simulink model "mdaqdemo_vs"  (R2013a)
settings: Solver=FixedStepDiscrete  StartTime=0.0  StopTime=inf  RelTol=1e-3
PreLoadFcn:
  | template_orig = fliplr([109 100]);
  | template_size = fliplr([18 22]);
  | search_border = fliplr([10 15]);
  | pos.template_orig = fliplr(template_orig);
  | pos.template_size = template_size;
  | pos.search_border = search_border;
  | pos.template_center = floor((template_size-1)/2);
  | pos.template_center_pos = pos.template_orig + ...
  |     pos.template_center - 1;
undefined symbols (not defined in the file or in its folder): gray
libraries: visiontextngfix x3, visionsinks x2, visiongeotforms x1, dspvision x1
Description:
  | Image stabilization demo.
settings Model: Tag="0  0  0  0  0  1"  FPTRunName=Active  ExtModeAutoUpdateStatusClock=off  Creator=The MathWorks Inc.  LastModifiedBy=witczenko
settings DataIOCC: SignalLoggingSaveFormat=ModelDataLogs  SaveOutput=off  SaveTime=off  SignalLoggingName=logsOut
settings OptimizationCC: InlineParams=on  ExpressionDepthLimit=2147483647  InitFltsAndDblsToZero=on  OptimizeModelRefInitCode=on  LifeSpan=Inf  BufferReusableBoundary=off
settings DebuggingCC: CheckExecutionContextPreStartOutputMsg=on  CheckExecutionContextRuntimeOutputMsg=on  SolverPrmCheckMsg=none  InheritedTsInSrcMsg=none  MultiTaskDSMMsg=warning  SigSpecEnsureSampleTimeMsg=none  ParameterPrecisionLossMsg=none  UnderSpecifiedDataTypeMsg=error  FcnCallInpInsideContextMsg=EnableAllAsWarning  FrameProcessingCompatibilityMsg=error  BusObjectLabelMismatch=none
settings HardwareCC: ProdBitPerLong=40  ProdLargestAtomicInteger=Integer  ProdIntDivRoundTo=Zero  ProdEndianess=LittleEndian  ProdHWDeviceType=Texas Instruments->C6000  TargetBitPerPointer=64  TargetLongLongMode=on  TargetIntDivRoundTo=Zero  TargetEndianess=LittleEndian  TargetWordSize=64  TargetHWDeviceType=MATLAB Host  ProdEqTarget=off
settings ModelReferenceCC: UpdateModelReferenceTargets=IfOutOfDate
settings RTWCC: SystemTargetFile=microdaq.tlc  TemplateMakefile=microdaq.tmf  PostCodeGenCommand=microdaq_postcodegen(buildInfo)  Description=MicroDAQ Real-Time Measurement System
settings CodeAppCC: IgnoreCustomStorageClasses=off
settings STFCustomTargetCC: CodeReplacementLibrary=C89/C90 (ANSI)  CombineOutputUpdateFcns=on  ERTCustomFileBanners=on  SupportContinuousTime=off  SupportNonInlinedSFcns=off  MATLABClassNameForMDSCustomization=Simulink.SoftwareTarget.ERTCustomization  SystemTargetFile=microdaq.tlc
settings ERTTargetCC: CodeReplacementLibrary=C89/C90 (ANSI)  GenerateSampleERTMain=off  ParMdlRefBuildCompliant=off  CompOptLevelCompliant=off  ConcurrentExecutionCompliant=off  ERTFirstTimeCompliant=off  ModelStepFunctionPrototypeControlCompliant=off  CPPClassGenCompliant=off  ERTCustomFileTemplate=microdaq_main.tlc

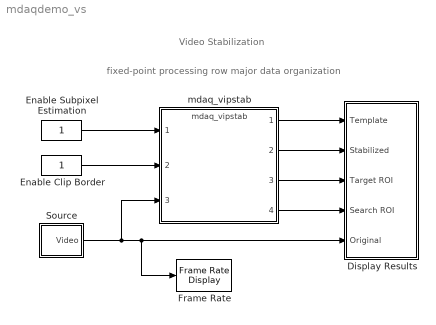
== system mdaqdemo_vs ==
  note: Video Stabilization
  note: fixed-point processing
      | row major data organization
  Display Results : Subsystem
  Enable Clip Border : Constant  VectorParams1D=off  OutDataTypeStr=boolean  SampleTime=-1
  Enable Subpixel Estimation : Constant  VectorParams1D=off  OutDataTypeStr=boolean  SampleTime=-1
  Frame Rate : visionsinks/Frame Rate Display  UpdateRate=10
  Source : Subsystem
  mdaq_vipstab : ModelReference  ModelNameDialog=mdaq_vipstab  SimulationMode=Processor-in-the-loop (PIL)  ModelReferenceVersion=1.1886
  wires:
  Source/1(Video) -> mdaq_vipstab/3, Frame Rate/1, Display Results/5(Original)
  mdaq_vipstab/1 -> Display Results/1(Template)
  mdaq_vipstab/2 -> Display Results/2(Stabilized)
  Enable Subpixel Estimation/1 -> mdaq_vipstab/1
  Enable Clip Border/1 -> mdaq_vipstab/2
  mdaq_vipstab/3 -> Display Results/3(Target ROI)
  mdaq_vipstab/4 -> Display Results/4(Search ROI)

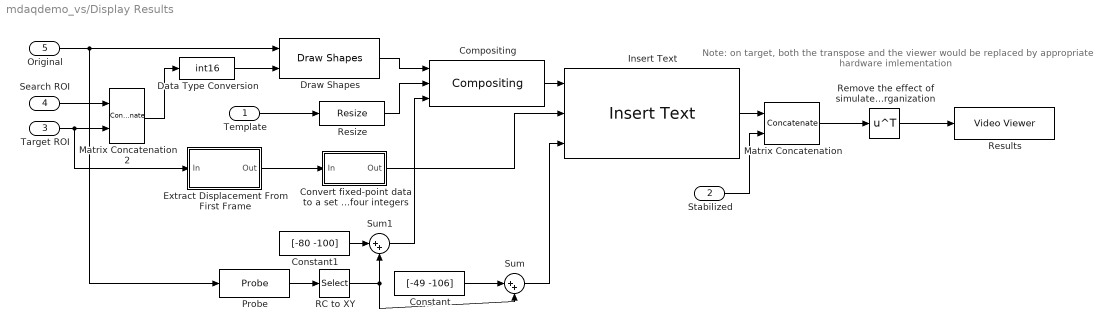
== system mdaqdemo_vs/Display Results ==
  note: Note: on target, both the transpose and the viewer
      | would be replaced by appropriate hardware imlementation
  Template : Inport
  Stabilized : Inport  Port=2
  Target ROI : Inport  Port=3
  Search ROI : Inport  Port=4
  Original : Inport  Port=5
  Compositing : visiontextngfix/Compositing  operation=Binary mask  bFacSrc=Specify via dialog  mFacSrc=Specify via dialog  bFactor=1  mFactor=1  source=Input port  coordinates=[160 220]  prodOutputMode=Binary point scaling  prodOutputWordLength=32  prodOutputFracLength=10  roundingMode=Floor  overflowMode=off
  Constant : Constant  Value=[-49 -106]  OutDataTypeStr=int16
  Constant1 : Constant  Value=[-80 -100]  OutDataTypeStr=int16
  Convert fixed-point data to a set of four integers : Subsystem
  Data Type Conversion : DataTypeConversion  OutDataTypeStr=int16
  Draw Shapes : visiontextngfix/Draw Shapes  shape=Rectangles  fill=off  fillClrSource=Specify via dialog  display=White  intensity=200  color=[200 255 100]  opacity=0.6  viewport=Entire image  antialiasing=off  inType=Intensity  imagePorts=One multidimensional signal  prodOutputMode=Binary point scaling  prodOutputWordLength=32  prodOutputFracLength=14  memoryMode=Specify word length  memoryWordLength=16  memoryFracLength=15  roundingMode=Floor  overflowMode=off
  Extract Displacement From First Frame : Subsystem
  Insert Text : visiontextngfix/Insert Text  inputType=Obsolete  theText='(%+03d.%02d,%+03d.%02d)'  fontFace=LucidaTypewriterRegular  dummyVar1=0  blockFontSize=14  antiAliased=on  getTextLocFrom=Input port  textLoc=[214 191]  getTextColorFrom=Specify via dialog  textColor=255  getTextIntensityFrom=Specify via dialog  textIntensity=255  getTextOpacityFrom=Specify via dialog  textOpacity=1.0  dummyVar2=0  dummyVar3=0  dummyVar4=0  imagePorts=One multidimensional signal  isInputTransposed=on
  Matrix Concatenation : Concatenate  Mode=Multidimensional array
  Matrix Concatenation2 : Concatenate  Mode=Multidimensional array
  Probe : Probe  ProbeWidth=off  ProbeSampleTime=off  ProbeComplexSignal=off  ProbeSignalDimensions=on  ProbeDimensionsDataType=int16
  RC to XY : Selector  IndexOptions=Index vector (dialog)  Indices=[2 1]  OutputSizes=1
  Remove the effect of simulated row major data organization : Math  Operator=transpose  SaturateOnIntegerOverflow=on
  Resize : visiongeotforms/Resize  specify=Output size as a percentage of input size  rfactor=300  outCols=25  outRows=25  outRowsCols=[25 35]  interp_method=Nearest neighbor  antialias=off  useROI=off  roiFlag=off  prodOutputMode=Binary point scaling  prodOutputWordLength=32  prodOutputFracLength=10  roundingMode=Nearest  overflowMode=on
  Results : visionsinks/Video Viewer  inputType=Obsolete7b  imagePorts=One multidimensional signal  useColorMap=off  colormapValue=gray(256)  specRange=off  minInputVal=0  maxInputVal=255  FigPos=[97 364 640 263]  AxisZoom=on  trueSizedOnce=on  OpenAtMdlStart=on  DefaultConfigurationName=vipscopes.VideoViewerScopeCfg
  Sum : Sum  Inputs=|++
  Sum1 : Sum  Inputs=|++
  wires:
  Remove the effect of simulated row major data organization/1 -> Results/1
  RC to XY/1 -> Sum/2, Sum1/2
  Constant/1 -> Sum/1
  Sum/1 -> Insert Text/3
  Probe/1 -> RC to XY/1
  Sum1/1 -> Compositing/3
  Constant1/1 -> Sum1/1
  Template/1 -> Resize/1
  Compositing/1 -> Insert Text/1
  Insert Text/1 -> Matrix Concatenation/1
  Resize/1 -> Compositing/2
  Stabilized/1 -> Matrix Concatenation/2
  Draw Shapes/1 -> Compositing/1
  Matrix Concatenation/1 -> Remove the effect of simulated row major data organization/1
  Convert fixed-point data to a set of four integers/1(Out) -> Insert Text/2
  Matrix Concatenation2/1 -> Data Type Conversion/1
  Original/1 -> Probe/1, Draw Shapes/1
  Extract Displacement From First Frame/1(Out) -> Convert fixed-point data to a set of four integers/1(In)
  Search ROI/1 -> Matrix Concatenation2/1
  Target ROI/1 -> Matrix Concatenation2/2, Extract Displacement From First Frame/1(In)
  Data Type Conversion/1 -> Draw Shapes/2

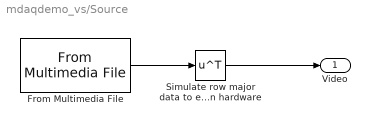
== system mdaqdemo_vs/Source ==
  From Multimedia File : dspvision/From Multimedia File  inputFilename=shaky_car.avi  loop=on  numPlays=inf  outputStreams=Video and audio  videoDataType=uint8  audioDataType=int16  inheritSampleTime=on  userDefinedSampleTime=1/30  noAudioOutput=off  isIntensityVideo=off  fourcc=Intensity  colorVideoFormat=Separate color signals  outputEOF=off  dataOrg=Column-major  audioFrameSize=1024  computeAudioFrameSize=off  outSamplingMode=Frame based
  Simulate row major data to ease implementation on hardware : Math  Operator=transpose  SaturateOnIntegerOverflow=on
  Video : Outport
  wires:
  Simulate row major data to ease implementation on hardware/1 -> Video/1
  From Multimedia File/1 -> Simulate row major data to ease implementation on hardware/1

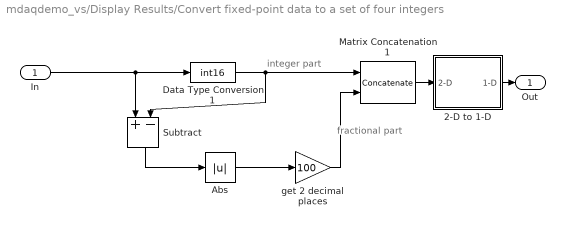
== system mdaqdemo_vs/Display Results/Convert fixed-point data to a set of four integers ==
  note: integer part
  note: fractional
      | part
  In : Inport
  2-D to 1-D : Subsystem
  Abs : Abs
  Data Type Conversion1 : DataTypeConversion  OutDataTypeStr=int16  RndMeth=Zero
  Matrix Concatenation1 : Concatenate  Mode=Multidimensional array
  Subtract : Sum  Inputs=+-  OutDataTypeStr=Inherit: Same as first input
  get 2 decimal places : Gain  Gain=100  OutDataTypeStr=fixdt(1,16,0)  SaturateOnIntegerOverflow=on
  Out : Outport
  wires:
  Matrix Concatenation1/1 -> 2-D to 1-D/1(2-D)
  Data Type Conversion1/1 -> Matrix Concatenation1/1, Subtract/2
  Subtract/1 -> Abs/1
  Abs/1 -> get 2 decimal places/1
  In/1 -> Data Type Conversion1/1, Subtract/1
  2-D to 1-D/1(1-D) -> Out/1
  get 2 decimal places/1 -> Matrix Concatenation1/2

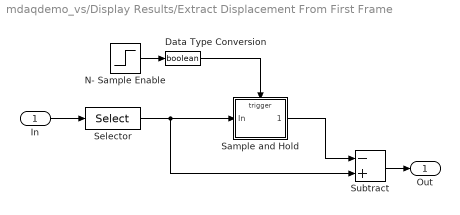
== system mdaqdemo_vs/Display Results/Extract Displacement From First Frame ==
  In : Inport
  Data Type Conversion : DataTypeConversion  OutDataTypeStr=boolean
  N- Sample Enable : Step  Time=0
  Sample and Hold : Subsystem  TreatAsAtomicUnit=on  mask{initCond=0}
      mask prompts: initCond "Initial Condition"
  Selector : Selector  NumberOfDimensions=2  InputPortWidth=3  IndexOptions=Index vector (dialog),Index vector (dialog)  Indices=1,[1 2]  OutputSizes=1,1
  Subtract : Sum  Inputs=-+
  Out : Outport
  wires:
  Data Type Conversion/1 -> Sample and Hold/Trigger
  In/1 -> Selector/1
  Selector/1 -> Subtract/2, Sample and Hold/1(In)
  Subtract/1 -> Out/1
  Sample and Hold/1(" ") -> Subtract/1
  N- Sample Enable/1 -> Data Type Conversion/1

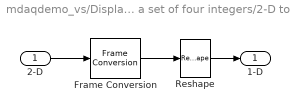
== system mdaqdemo_vs/Display Results/Convert fixed-point data to a set of four integers/2-D to 1-D ==
  2-D : Inport
  Frame Conversion : FrameConversion  InheritSamplingMode=off  OutFrame=Sample-based
  Reshape : Reshape
  1-D : Outport
  wires:
  2-D/1 -> Frame Conversion/1
  Frame Conversion/1 -> Reshape/1
  Reshape/1 -> 1-D/1

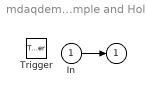
== system mdaqdemo_vs/Display Results/Extract Displacement From First Frame/Sample and Hold ==
  In : Inport
  Trigger : TriggerPort  ZeroCross=off
  " " : Outport  InitialOutput=initCond
  wires:
  In/1 -> " "/1
